simulink model "washing_machine"  (R2024b)
settings: Solver=VariableStepAuto  StartTime=0.0  StopTime=500  RelTol=1e-3
settings Model: Creator=Latitude E5300  LastModifiedBy=Latitude E5300

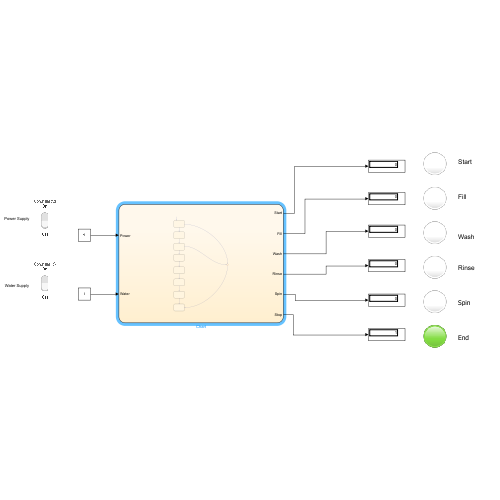
[thumbnail: Simulink's stored preview of the top-level diagram]
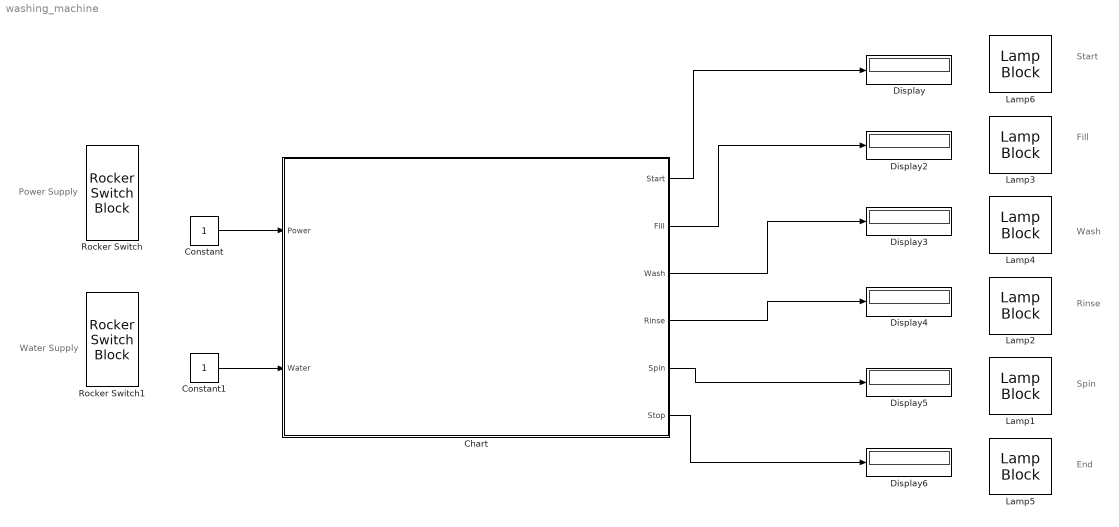
== system washing_machine ==
  note: Power Supply
  note: Water Supply
  note: Rinse
  note: Start
  note: Spin
  note: Wash
  note: End
  note: Fill
  Chart : Stateflow chart  TreatAsAtomicUnit=on
  Constant : Constant
  Constant1 : Constant
  Display{,2..6} (6 alike) : Display
  Lamp{1..6} (6 alike) : LampBlock  LabelPosition=Hide
  Rocker Switch : RockerSwitchBlock
      settings: Values={{'Off', 'On'}, [0 1]}
  Rocker Switch1 : RockerSwitchBlock
      settings: Values={{'Off', 'On'}, [0 1]}
  wires:
  Constant/1 -> Chart/1(Power)
  Constant1/1 -> Chart/2(Water)
  Chart/5(Spin) -> Display5/1
  Chart/6(Stop) -> Display6/1
  Chart/4(Rinse) -> Display4/1
  Chart/3(Wash) -> Display3/1
  Chart/2(Fill) -> Display2/1
  Chart/1(Start) -> Display/1

== stateflow chart washing_machine/Chart ==
  state Power
  state ON
    entry:Start=1
  state Water_Supply
  state FILL
    entry:Start=0;
    during:Fill=1;
  state WASH
    entry:Fill=0;
    during:Wash=0;
  state RINSE
    entry:Wash=0;
    during:Rinse=1;
  state SPIN
    entry:Rinse=0;
    during:Spin=1;
  state OFF
    entry:Spin=0;
    during:Stop=1
  (default) -> Power
  Power -> (junction 18) [order 2] : [Power==0]
  Power -> ON [order 1] : [Power==1]
  ON -> Water_Supply
  Water_Supply -> (junction 18) [order 2] : [Water==0]
  Water_Supply -> FILL [order 1] : [Water==1]
  FILL -> WASH : [after(200,sec)]
  (junction 18) -> OFF
  WASH -> RINSE : [after(100,sec)]
  RINSE -> SPIN : [after(20,sec)]
  SPIN -> OFF : [after(50,sec)]
  data: Power input; Water input; Start output; Fill output; Wash output; Rinse output; Spin output; Stop output
